simulink model "test_link_mux_demux"  (Simulink 7.3)
settings: Solver=ode45  StartTime=0.0  StopTime=100  RelTol=1e-3
undefined symbols (not defined in the file): ROACH
libraries: xbsIndex_r4 x46, xps_library x9, isi_correlator_lib x6, casper_library x1
settings Model: Creator=wjm  LastModifiedBy=wjm
settings OptimizationCC: InitFltsAndDblsToZero=on

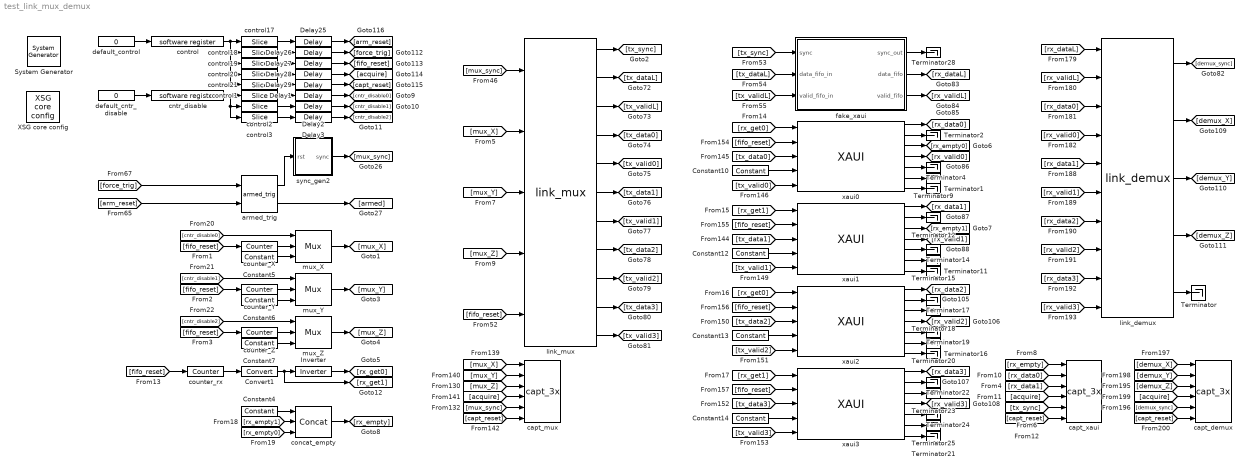
== system test_link_mux_demux ==
  " System Generator" : xbsIndex_r4/ System Generator  Tag=genX  SystemSampleTime=-1  xilinxfamily=virtex5  part=xc5vsx95t  speed=-1  package=ff1136  synthesis_tool=XST  clock_wrapper=Clock Enables  directory=./test_link_mux_demux/sysgen  testbench=off  simulink_period=1  sysclk_period=5  dcm_input_clock_period=100  incr_netlist=off  trim_vbits=Everywhere in SubSystem  dbl_ovrd=According to Block Masks  core_generation=According to Block Masks  run_coregen=off  deprecated_control=off  eval_field=0  block_type=sysgen
      settings: block_version=10.1.1
  Constant{10,12..14} (4 alike) : xbsIndex_r4/Constant  arith_type=Unsigned  const=0  n_bits=8  bin_pt=0  explicit_period=on  period=1  equ=P=C  opselect=C  inp2=PCIN>>17  opr=+  inp1=P  carry=CIN  dbl_ovrd=off  block_type=constant
      settings: block_version=10.1.1
  Constant{4..7} (4 alike) : xbsIndex_r4/Constant  arith_type=Unsigned  const=0  n_bits=30  bin_pt=0  explicit_period=on  period=1  equ=P=C  opselect=C  inp2=PCIN>>17  opr=+  inp1=P  carry=CIN  dbl_ovrd=off  block_type=constant
      settings: block_version=10.1.1
  Convert1 : xbsIndex_r4/Convert  arith_type=Boolean  n_bits=1  bin_pt=0  quantization=Truncate  overflow=Wrap  latency=3  dbl_ovrd=off  pipeline=on  block_type=convert
      settings: block_version=10.1.3
  Delay{1..3,25..29} (8 alike) : xbsIndex_r4/Delay  en=off  latency=3  dbl_ovrd=off  reg_retiming=off  block_type=delay
  Inverter : xbsIndex_r4/Inverter  en=off  latency=0  dbl_ovrd=off  block_type=inv
      settings: block_version=11.3
  Terminator{,1..2,4,9,11..12,14..25,28} (20 alike) : Terminator
  XSG core config : xps_library/XSG core config  Tag=xps:xsg  SystemSampleTime=-1  hw_sys=ROACH:sx95t  ibob_linux=off  clk_src=sys_clk2x  iBOB_clk_src=sys_clk  BEE2_ctrl_clk_src=sys_clk  BEE2_usr_clk_src=sys_clk  ROACH_clk_src=sys_clk2x  CORR_clk_src=sys_clk  gpio_clk_io_group=iBOB:sma  gpio_clk_bit_index=0  clk_rate=200  sample_period=1  synthesis_tool=XST  mpc_type=powerpc440_ext
  armed_trig : isi_correlator_lib/armed_trig  SystemSampleTime=-1
  capt_demux : isi_correlator_lib/capt_3x  SystemSampleTime=-1
      link override bram0/convert_din: arith_type=Unsigned
      link override bram0/mem/sim_data_in: arith_type=Unsigned
      link override bram0/test_link_mux_demux_capt_demux_bram0_data_out: arith_type=Unsigned
      link override bram1/convert_din: arith_type=Unsigned
      link override bram1/mem/sim_data_in: arith_type=Unsigned
      link override bram1/test_link_mux_demux_capt_demux_bram1_data_out: arith_type=Unsigned
      link override bram2/convert_din: arith_type=Unsigned
      link override bram2/mem/sim_data_in: arith_type=Unsigned
      link override bram2/test_link_mux_demux_capt_demux_bram2_data_out: arith_type=Unsigned
  capt_mux : isi_correlator_lib/capt_3x  SystemSampleTime=-1
      link override bram0/convert_din: arith_type=Unsigned
      link override bram0/mem/sim_data_in: arith_type=Unsigned
      link override bram0/test_link_mux_demux_capt_mux_bram0_data_out: arith_type=Unsigned
      link override bram1/convert_din: arith_type=Unsigned
      link override bram1/mem/sim_data_in: arith_type=Unsigned
      link override bram1/test_link_mux_demux_capt_mux_bram1_data_out: arith_type=Unsigned
      link override bram2/convert_din: arith_type=Unsigned
      link override bram2/mem/sim_data_in: arith_type=Unsigned
      link override bram2/test_link_mux_demux_capt_mux_bram2_data_out: arith_type=Unsigned
  capt_xaui : isi_correlator_lib/capt_3x  SystemSampleTime=-1
      link override bram0/convert_din: arith_type=Unsigned
      link override bram0/mem/sim_data_in: arith_type=Unsigned
      link override bram0/test_link_mux_demux_capt_demux_bram0_data_out: arith_type=Unsigned
      link override bram1/convert_din: arith_type=Unsigned
      link override bram1/mem/sim_data_in: arith_type=Unsigned
      link override bram1/test_link_mux_demux_capt_demux_bram1_data_out: arith_type=Unsigned
      link override bram2/convert_din: arith_type=Unsigned
      link override bram2/mem/sim_data_in: arith_type=Unsigned
      link override bram2/test_link_mux_demux_capt_demux_bram2_data_out: arith_type=Unsigned
  cntr_disable : xps_library/software register  Tag=xps:sw_reg  SystemSampleTime=-1  io_dir=From Processor  arith_type=Unsigned  bitwidth=32  bin_pt=0  sample_period=1  gw_name=test_link_mux_demux_cntr_disable_user_data_out
      link override corr_3ghz_10_1_corr_id_user_data_out: arith_type=Unsigned  n_bits=32  bin_pt=0  period=1
      link override corr_3ghz_10_1_exp_corr_id_user_data_out: arith_type=Unsigned  n_bits=32  bin_pt=0  period=1
      link override isi_corr_eq_coeff_user_data_out: arith_type=Unsigned  n_bits=32  bin_pt=0  period=1
      link override isi_correlator_control_user_data_out: arith_type=Unsigned  n_bits=32  bin_pt=0  period=1
      link override isi_correlator_cropped_control_user_data_out: arith_type=Unsigned  n_bits=32  bin_pt=0  period=1
      link override isi_correlator_eq_coeff_user_data_out: arith_type=Unsigned  n_bits=32  bin_pt=0  period=1
      link override isi_spectrometer_control_user_data_out: arith_type=Unsigned  n_bits=32  bin_pt=0  period=1
      link override isi_spectrometer_cropped_control_user_data_out: arith_type=Unsigned  n_bits=32  bin_pt=0  period=1
      link override isi_spectrometer_with_pfb_control_user_data_out: arith_type=Unsigned  n_bits=32  bin_pt=0  period=1
      link override roach_spectrometer_control_user_data_out: arith_type=Unsigned  n_bits=32  bin_pt=0  period=1
      link override test_link_mux_demux_control_user_data_out: arith_type=Unsigned  n_bits=32  bin_pt=0  period=1
  concat_empty : xbsIndex_r4/Concat  num_inputs=3  dbl_ovrd=off  block_type=concat
      settings: block_version=10.1.1
  control : xps_library/software register  Tag=xps:sw_reg  SystemSampleTime=-1  io_dir=From Processor  arith_type=Unsigned  bitwidth=32  bin_pt=0  sample_period=1  gw_name=test_link_mux_demux_control_user_data_out
      link override corr_3ghz_10_1_corr_id_user_data_out: arith_type=Unsigned  n_bits=32  bin_pt=0  period=1
      link override corr_3ghz_10_1_exp_corr_id_user_data_out: arith_type=Unsigned  n_bits=32  bin_pt=0  period=1
      link override isi_corr_eq_coeff_user_data_out: arith_type=Unsigned  n_bits=32  bin_pt=0  period=1
      link override isi_correlator_control_user_data_out: arith_type=Unsigned  n_bits=32  bin_pt=0  period=1
      link override isi_correlator_cropped_control_user_data_out: arith_type=Unsigned  n_bits=32  bin_pt=0  period=1
      link override isi_correlator_eq_coeff_user_data_out: arith_type=Unsigned  n_bits=32  bin_pt=0  period=1
      link override isi_spectrometer_control_user_data_out: arith_type=Unsigned  n_bits=32  bin_pt=0  period=1
      link override isi_spectrometer_cropped_control_user_data_out: arith_type=Unsigned  n_bits=32  bin_pt=0  period=1
      link override isi_spectrometer_with_pfb_control_user_data_out: arith_type=Unsigned  n_bits=32  bin_pt=0  period=1
      link override roach_spectrometer_control_user_data_out: arith_type=Unsigned  n_bits=32  bin_pt=0  period=1
      link override test_link_mux_demux_control_user_data_out: arith_type=Unsigned  n_bits=32  bin_pt=0  period=1
  control1 : xbsIndex_r4/Slice  nbits=1  boolean_output=off  mode=Lower Bit Location + Width  bit1=0  base1=MSB of Input  bit0=0  base0=LSB of Input  dbl_ovrd=off  block_type=slice
      settings: block_version=10.1.3
  control17 : xbsIndex_r4/Slice  nbits=1  boolean_output=on  mode=Lower Bit Location + Width  bit1=0  base1=MSB of Input  bit0=0  base0=LSB of Input  dbl_ovrd=off  block_type=slice
      settings: infoedit="Extracts a given range of bits from each input sample and presents it at the output.  The output type is ordinarily unsigned with binary point at zero, but can be Boolean when the slice is one bit wide.<P><P>Hardware notes: In hardware this block costs nothing."  block_version=10.1.3
  control18 : xbsIndex_r4/Slice  nbits=1  boolean_output=on  mode=Lower Bit Location + Width  bit1=0  base1=MSB of Input  bit0=1  base0=LSB of Input  dbl_ovrd=off  block_type=slice
      settings: infoedit="Extracts a given range of bits from each input sample and presents it at the output.  The output type is ordinarily unsigned with binary point at zero, but can be Boolean when the slice is one bit wide.<P><P>Hardware notes: In hardware this block costs nothing."  block_version=10.1.3
  control19 : xbsIndex_r4/Slice  nbits=1  boolean_output=on  mode=Lower Bit Location + Width  bit1=0  base1=MSB of Input  bit0=2  base0=LSB of Input  dbl_ovrd=off  block_type=slice
      settings: infoedit="Extracts a given range of bits from each input sample and presents it at the output.  The output type is ordinarily unsigned with binary point at zero, but can be Boolean when the slice is one bit wide.<P><P>Hardware notes: In hardware this block costs nothing."  block_version=10.1.3
  control2 : xbsIndex_r4/Slice  nbits=1  boolean_output=off  mode=Lower Bit Location + Width  bit1=0  base1=MSB of Input  bit0=1  base0=LSB of Input  dbl_ovrd=off  block_type=slice
      settings: block_version=10.1.3
  control20 : xbsIndex_r4/Slice  nbits=1  boolean_output=on  mode=Lower Bit Location + Width  bit1=0  base1=MSB of Input  bit0=3  base0=LSB of Input  dbl_ovrd=off  block_type=slice
      settings: infoedit="Extracts a given range of bits from each input sample and presents it at the output.  The output type is ordinarily unsigned with binary point at zero, but can be Boolean when the slice is one bit wide.<P><P>Hardware notes: In hardware this block costs nothing."  block_version=10.1.3
  control21 : xbsIndex_r4/Slice  nbits=1  boolean_output=on  mode=Lower Bit Location + Width  bit1=0  base1=MSB of Input  bit0=4  base0=LSB of Input  dbl_ovrd=off  block_type=slice
      settings: infoedit="Extracts a given range of bits from each input sample and presents it at the output.  The output type is ordinarily unsigned with binary point at zero, but can be Boolean when the slice is one bit wide.<P><P>Hardware notes: In hardware this block costs nothing."  block_version=10.1.3
  control3 : xbsIndex_r4/Slice  nbits=1  boolean_output=off  mode=Lower Bit Location + Width  bit1=0  base1=MSB of Input  bit0=2  base0=LSB of Input  dbl_ovrd=off  block_type=slice
      settings: block_version=10.1.3
  counter_X : xbsIndex_r4/Counter  cnt_type=Free Running  cnt_to=Inf  operation=Up  start_count=0  cnt_by_val=1  arith_type=Unsigned  n_bits=30  bin_pt=0  load_pin=off  rst=on  en=off  explicit_period=on  period=1  dbl_ovrd=off  use_behavioral_HDL=off  implementation=Fabric  use_rpm=off  block_type=counter
  counter_Y : xbsIndex_r4/Counter  cnt_type=Free Running  cnt_to=Inf  operation=Up  start_count=0  cnt_by_val=1  arith_type=Unsigned  n_bits=30  bin_pt=0  load_pin=off  rst=on  en=off  explicit_period=on  period=1  dbl_ovrd=off  use_behavioral_HDL=off  implementation=Fabric  use_rpm=off  block_type=counter
  counter_Z : xbsIndex_r4/Counter  cnt_type=Free Running  cnt_to=Inf  operation=Up  start_count=0  cnt_by_val=1  arith_type=Unsigned  n_bits=30  bin_pt=0  load_pin=off  rst=on  en=off  explicit_period=on  period=1  dbl_ovrd=off  use_behavioral_HDL=off  implementation=Fabric  use_rpm=off  block_type=counter
  counter_rx : xbsIndex_r4/Counter  cnt_type=Free Running  cnt_to=Inf  operation=Up  start_count=0  cnt_by_val=1  arith_type=Unsigned  n_bits=1  bin_pt=0  load_pin=off  rst=on  en=off  explicit_period=on  period=1  dbl_ovrd=off  use_behavioral_HDL=off  implementation=Fabric  use_rpm=off  block_type=counter
  default_cntr_disable : Constant  Value=0  OutDataType=sfix(16)  OutScaling=2^0  SampleTime=1
  default_control : Constant  Value=0  OutDataType=sfix(16)  OutScaling=2^0  SampleTime=1
  fake_xaui : Subsystem  AncestorBlock=isi_correlator_lib/fake_xaui  mask{latency=64}
  link_demux : isi_correlator_lib/link_demux  SystemSampleTime=-1  buffer_depth=8  logic_latency=1  mux_latency=1
  link_mux : isi_correlator_lib/link_mux  SystemSampleTime=-1
  mux_X : xbsIndex_r4/Mux  inputs=2  en=off  latency=0  precision=Full  arith_type=Unsigned  n_bits=16  bin_pt=14  quantization=Truncate  overflow=Wrap  dbl_ovrd=off  block_type=mux
      settings: block_version=11.3
  mux_Y : xbsIndex_r4/Mux  inputs=2  en=off  latency=0  precision=Full  arith_type=Unsigned  n_bits=16  bin_pt=14  quantization=Truncate  overflow=Wrap  dbl_ovrd=off  block_type=mux
      settings: block_version=11.3
  mux_Z : xbsIndex_r4/Mux  inputs=2  en=off  latency=0  precision=Full  arith_type=Unsigned  n_bits=16  bin_pt=14  quantization=Truncate  overflow=Wrap  dbl_ovrd=off  block_type=mux
      settings: block_version=11.3
  sync_gen2 : Subsystem  AncestorBlock=isi_correlator_lib/sync_gen2  mask(sync_gen2){using_pfb_fir=off, pfb_fir_taps=4, using_fft=off, fft_size=7, fft_inputs=4, fft_orders=[2 2 2 1], using_ct=off, ct_type=Double-buffered, using_vacc=off, vacc_length=0, using_scale_factor=on, scale_factor=2^20}
      mask prompts: using_pfb_fir "This design uses a PFB FIR."; pfb_fir_taps "Number of taps in PFB FIR:"; using_fft "This design uses an FFT."; fft_size "Size of FFT: (2^?)"; fft_inputs "Number of FFT inputs: (2^?)"; fft_orders "Order of FFT reorders: (vector)"; using_ct "This design uses a corner turner."; ct_type "Type of reorder operation:"; using_vacc "This design uses a vector accumulator."; vacc_length "Length of accumulations: (2^?)"; using_scale_factor "Scale the minimum period by an arbitrary amount."; scale_factor "Scale factor:"
      mask help: This block generates a sync pulse of an appropriate period based on the specified mask parameters.
      mask init:
      | sync_gen2_init(gcb, ...
      |     'using_pfb_fir', using_pfb_fir, ...
      |     'pfb_fir_taps', pfb_fir_taps, ...
      |     'using_fft', using_fft, ...
      |     'fft_size', fft_size, ...
      |     'fft_inputs', fft_inputs, ...
      |     'fft_orders', fft_orders, ...
      |     'using_ct', using_ct, ...
      |     'ct_type', ct_type, ...
      |     'using_vacc', using_vacc, ...
      |     'vacc_length', vacc_length, ...
      |     'using_scale_factor', using_scale_factor, ...
      |     'scale_factor', scale_factor);
      settings: AttributesFormatString=sync_period=1048576
      mask StyleString: checkbox,edit,checkbox,edit,edit,edit,checkbox,popup(Double-buffered|In-place),checkbox,edit,checkbox,edit
      mask CallbackString:
      | thisVariable = 'using_pfb_fir';
      | affectedVars = {'pfb_fir_taps'};
      | 
      | thisBlock = gcb();
      | thisVarState = get_param(thisBlock, thisVariable);
      | maskNames = get_param(thisBlock, 'MaskNames');
      | maskEnables = get_param(thisBlock, 'MaskEnables');
      | 
      | for varName = affectedVars
      |     varIndex = find(ismember(maskNames, varName));
      |     maskEnables{varIndex} = thisVarState;
      | end
      | 
      | set_param(thisBlock, 'MaskEnables', maskEnables);||thisVariable = 'using_fft';
      | affectedVars = {'fft_size', 'fft_inputs', 'fft_orders'};
      | 
      | thisBlock = gcb();
      | thisVarState = get_param(thisBlock, thisVariable);
      | maskNames = get_param(thisBlock, 'MaskNames');
      | maskEnables = get_param(thisBlock, 'MaskEnables');
      | 
      | for varName = affectedVars
      |     varIndex = find(ismember(maskNames, varName));
      |     maskEnables{varIndex} = thisVarState;
      | end
      | 
      | set_param(thisBlock, 'MaskEnables', maskEnables);||||thisVariable = 'using_ct';
      | affectedVars = {'ct_type'};
      | 
      | thisBlock = gcb();
      | thisVarState = get_param(thisBlock, thisVariable);
      | maskNames = get_param(thisBlock, 'MaskNames');
      | maskEnables = get_param(thisBlock, 'MaskEnables');
      | 
      | for varName = affectedVars
      |     varIndex = find(ismember(maskNames, varName));
      |     maskEnables{varIndex} = thisVarState;
      | end
      | 
      | set_param(thisBlock, 'MaskEnables', maskEnables);||thisVariable = 'using_vacc';
      | affectedVars = {'vacc_length'};
      | 
      | thisBlock = gcb();
      | thisVarState = get_param(thisBlock, thisVariable);
      | maskNames = get_param(thisBlock, 'MaskNames');
      | maskEnables = get_param(thisBlock, 'MaskEnables');
      | 
      | for varName = affectedVars
      |     varIndex = find(ismember(maskNames, varName));
      |     maskEnables{varIndex} = thisVarState;
      | end
      | 
      | set_param(thisBlock, 'MaskEnables', maskEnables);||thisVariable = 'using_scale_factor';
      | affectedVars = {'scale_factor'};
      | 
      | thisBlock = gcb();
      | thisVarState = get_param(thisBlock, thisVariable);
      | maskNames = get_param(thisBlock, 'MaskNames');
      | maskEnables = get_param(thisBlock, 'MaskEnables');
      | 
      | for varName = affectedVars
      |     varIndex = find(ismember(maskNames, varName));
      |     maskEnables{varIndex} = thisVarState;
      | end
      | 
      | set_param(thisBlock, 'MaskEnables', maskEnables);|
  xaui0 : xps_library/XAUI  Tag=xps:xaui  SystemSampleTime=-1  demux=2  port=ROACH:0  open_phy=on  show_param=off  pre_emph=3  swing=800
      link override convert_tx_data: n_bits=32
      link override convert_tx_outofband: n_bits=4
      link override test_link_mux_demux_xaui0_rx_data: n_bits=32
      link override test_link_mux_demux_xaui0_rx_outofband: n_bits=4
  xaui1 : xps_library/XAUI  Tag=xps:xaui  SystemSampleTime=-1  demux=2  port=ROACH:1  open_phy=on  show_param=off  pre_emph=3  swing=800
      link override convert_tx_data: n_bits=32
      link override convert_tx_outofband: n_bits=4
      link override test_link_mux_demux_xaui1_rx_data: n_bits=32
      link override test_link_mux_demux_xaui1_rx_outofband: n_bits=4
  xaui2 : xps_library/XAUI  Tag=xps:xaui  SystemSampleTime=-1  demux=2  port=ROACH:2  open_phy=on  show_param=off  pre_emph=3  swing=800
      link override convert_tx_data: n_bits=32
      link override convert_tx_outofband: n_bits=4
      link override test_link_mux_demux_xaui2_rx_data: n_bits=32
      link override test_link_mux_demux_xaui2_rx_outofband: n_bits=4
  xaui3 : xps_library/XAUI  Tag=xps:xaui  SystemSampleTime=-1  demux=2  port=ROACH:3  open_phy=on  show_param=off  pre_emph=3  swing=800
      link override convert_tx_data: n_bits=32
      link override convert_tx_outofband: n_bits=4
      link override test_link_mux_demux_xaui3_rx_data: n_bits=32
      link override test_link_mux_demux_xaui3_rx_outofband: n_bits=4
  wires:
  [mux_X] -> capt_mux/1
  [mux_Y] -> capt_mux/2
  [mux_Z] -> capt_mux/3
  [capt_reset] -> capt_mux/6
  [fifo_reset] -> link_mux/5
  link_mux/1 -> [tx_sync]
  link_mux/2 -> [tx_dataL]
  link_mux/3 -> [tx_validL]
  link_mux/4 -> [tx_data0]
  link_mux/5 -> [tx_valid0]
  link_mux/6 -> [tx_data1]
  link_mux/7 -> [tx_valid1]
  link_mux/8 -> [tx_data2]
  link_mux/9 -> [tx_valid2]
  link_mux/10 -> [tx_data3]
  link_mux/11 -> [tx_valid3]
  [tx_sync] -> fake_xaui/1(sync)
  [tx_dataL] -> fake_xaui/2(data_fifo_in)
  [tx_validL] -> fake_xaui/3(valid_fifo_in)
  [fifo_reset] -> xaui0/2
  [tx_data0] -> xaui0/3
  Constant10/1 -> xaui0/4
  [tx_valid0] -> xaui0/5
  [fifo_reset] -> xaui1/2
  [tx_data1] -> xaui1/3
  Constant12/1 -> xaui1/4
  [tx_valid1] -> xaui1/5
  [fifo_reset] -> xaui2/2
  [tx_data2] -> xaui2/3
  Constant13/1 -> xaui2/4
  [tx_valid2] -> xaui2/5
  [fifo_reset] -> xaui3/2
  [tx_data3] -> xaui3/3
  Constant14/1 -> xaui3/4
  [tx_valid3] -> xaui3/5
  xaui0/1 -> [rx_data0]
  xaui0/2 -> Terminator2/1
  xaui0/3 -> [rx_empty0]
  xaui0/4 -> [rx_valid0]
  xaui0/5 -> Terminator4/1
  xaui0/6 -> Terminator9/1
  xaui0/7 -> Terminator1/1
  xaui1/1 -> [rx_data1]
  xaui1/2 -> Terminator12/1
  xaui1/3 -> [rx_empty1]
  xaui1/4 -> [rx_valid1]
  xaui1/5 -> Terminator14/1
  xaui1/6 -> Terminator15/1
  xaui1/7 -> Terminator11/1
  xaui2/1 -> [rx_data2]
  xaui2/2 -> Terminator17/1
  xaui2/3 -> Terminator18/1
  xaui2/4 -> [rx_valid2]
  xaui2/5 -> Terminator19/1
  xaui2/6 -> Terminator20/1
  xaui2/7 -> Terminator16/1
  xaui3/1 -> [rx_data3]
  xaui3/2 -> Terminator22/1
  xaui3/3 -> Terminator23/1
  xaui3/4 -> [rx_valid3]
  xaui3/5 -> Terminator24/1
  xaui3/6 -> Terminator25/1
  xaui3/7 -> Terminator21/1
  fake_xaui/2(data_fifo) -> [rx_dataL]
  fake_xaui/3(valid_fifo) -> [rx_validL]
  [acquire] -> capt_mux/4
  [mux_sync] -> capt_mux/5
  fake_xaui/1(sync_out) -> Terminator28/1
  [demux_Y] -> capt_demux/2
  [demux_Z] -> capt_demux/3
  [capt_reset] -> capt_demux/6
  [acquire] -> capt_demux/4
  [demux_sync] -> capt_demux/5
  [arm_reset] -> armed_trig/2
  [force_trig] -> armed_trig/1
  armed_trig/1 -> sync_gen2/1(rst)
  armed_trig/2 -> [armed]
  sync_gen2/1(sync) -> [mux_sync]
  control21/1 -> Delay29/1
  control20/1 -> Delay28/1
  control19/1 -> Delay27/1
  control18/1 -> Delay26/1
  control17/1 -> Delay25/1
  control/1 -> control17/1, control18/1, control19/1, control21/1, control20/1
  Delay26/1 -> [force_trig]
  Delay27/1 -> [fifo_reset]
  Delay28/1 -> [acquire]
  Delay29/1 -> [capt_reset]
  default_control/1 -> control/1
  Delay25/1 -> [arm_reset]
  [mux_sync] -> link_mux/1
  [rx_dataL] -> link_demux/1
  [rx_validL] -> link_demux/2
  [rx_data0] -> link_demux/3
  [rx_valid0] -> link_demux/4
  [rx_data1] -> link_demux/5
  [rx_valid1] -> link_demux/6
  [rx_data2] -> link_demux/7
  [rx_valid2] -> link_demux/8
  [rx_data3] -> link_demux/9
  [rx_valid3] -> link_demux/10
  link_demux/5 -> Terminator/1
  link_demux/4 -> [demux_Z]
  link_demux/3 -> [demux_Y]
  link_demux/2 -> [demux_X]
  link_demux/1 -> [demux_sync]
  [demux_X] -> capt_demux/1
  [fifo_reset] -> counter_X/1
  [fifo_reset] -> counter_Y/1
  [fifo_reset] -> counter_Z/1
  [rx_data0] -> capt_xaui/2
  [rx_data1] -> capt_xaui/3
  [capt_reset] -> capt_xaui/6
  [acquire] -> capt_xaui/4
  [tx_sync] -> capt_xaui/5
  [rx_empty] -> capt_xaui/1
  [fifo_reset] -> counter_rx/1
  counter_rx/1 -> Convert1/1
  [rx_get0] -> xaui0/1
  [rx_get1] -> xaui1/1
  [rx_get0] -> xaui2/1
  [rx_get1] -> xaui3/1
  Constant4/1 -> concat_empty/1
  [rx_empty1] -> concat_empty/2
  [rx_empty0] -> concat_empty/3
  concat_empty/1 -> [rx_empty]
  default_cntr_disable/1 -> cntr_disable/1
  mux_X/1 -> [mux_X]
  mux_Y/1 -> [mux_Y]
  mux_Z/1 -> [mux_Z]
  counter_Z/1 -> mux_Z/2
  Constant7/1 -> mux_Z/3
  Constant6/1 -> mux_Y/3
  counter_Y/1 -> mux_Y/2
  Constant5/1 -> mux_X/3
  counter_X/1 -> mux_X/2
  cntr_disable/1 -> control1/1, control3/1, control2/1
  control1/1 -> Delay1/1
  Delay1/1 -> [cntr_disable0]
  [cntr_disable0] -> mux_X/1
  [cntr_disable1] -> mux_Y/1
  [cntr_disable2] -> mux_Z/1
  Convert1/1 -> Inverter/1, [rx_get1]
  control2/1 -> Delay2/1
  Delay2/1 -> [cntr_disable1]
  control3/1 -> Delay3/1
  Delay3/1 -> [cntr_disable2]
  [mux_Y] -> link_mux/3
  [mux_Z] -> link_mux/4
  [mux_X] -> link_mux/2
  Inverter/1 -> [rx_get0]

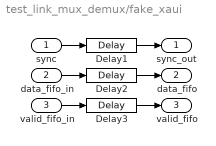
== system test_link_mux_demux/fake_xaui ==
  sync : Inport  OutDataType=sfix(16)  OutScaling=2^0
  data_fifo_in : Inport  Port=2  OutDataType=sfix(16)  OutScaling=2^0
  valid_fifo_in : Inport  Port=3  OutDataType=sfix(16)  OutScaling=2^0
  Delay1 : xbsIndex_r4/Delay  en=off  latency=latency  dbl_ovrd=off  reg_retiming=off  block_type=delay
  Delay2 : xbsIndex_r4/Delay  en=off  latency=latency  dbl_ovrd=off  reg_retiming=off  block_type=delay
  Delay3 : xbsIndex_r4/Delay  en=off  latency=latency  dbl_ovrd=off  reg_retiming=off  block_type=delay
  sync_out : Outport  OutDataType=sfix(16)  OutScaling=2^0
  data_fifo : Outport  Port=2  OutDataType=sfix(16)  OutScaling=2^0
  valid_fifo : Outport  Port=3  OutDataType=sfix(16)  OutScaling=2^0
  wires:
  valid_fifo_in/1 -> Delay3/1
  data_fifo_in/1 -> Delay2/1
  sync/1 -> Delay1/1
  Delay1/1 -> sync_out/1
  Delay2/1 -> data_fifo/1
  Delay3/1 -> valid_fifo/1

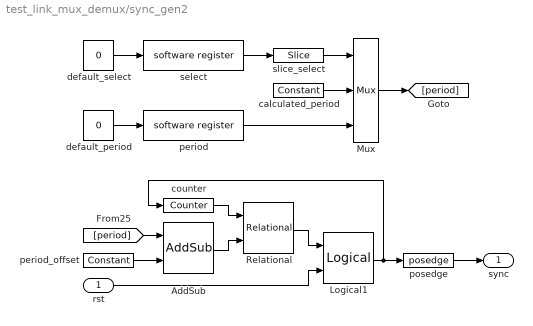
== system test_link_mux_demux/sync_gen2 ==
  rst : Inport  OutDataType=sfix(16)  OutScaling=2^0
  AddSub : xbsIndex_r4/AddSub  mode=Subtraction  use_carryin=off  use_carryout=off  en=off  latency=2  precision=Full  arith_type=Unsigned  n_bits=16  bin_pt=14  quantization=Truncate  overflow=Wrap  dbl_ovrd=off  use_behavioral_HDL=off  hw_selection=Fabric  pipelined=off  use_rpm=on  block_type=addsub
      settings: block_version=10.1.3
  Logical1 : xbsIndex_r4/Logical  logical_function=OR  inputs=2  en=off  latency=0  precision=Full  arith_type=Unsigned  n_bits=16  bin_pt=0  align_bp=on  dbl_ovrd=off  block_type=logical
  Mux : xbsIndex_r4/Mux  inputs=2  en=off  latency=0  precision=Full  arith_type=Unsigned  n_bits=16  bin_pt=14  quantization=Truncate  overflow=Wrap  dbl_ovrd=off  block_type=mux
  Relational : xbsIndex_r4/Relational  mode=a>=b  en=off  latency=1  dbl_ovrd=off  block_type=relational
      settings: block_version=10.1.3
  calculated_period : xbsIndex_r4/Constant  arith_type=Unsigned  const=1048576  n_bits=32  bin_pt=0  explicit_period=on  period=1  equ=P=C  opselect=C  inp2=PCIN>>17  opr=+  inp1=P  carry=CIN  dbl_ovrd=off  block_type=constant
      settings: block_version=10.1.1
  counter : xbsIndex_r4/Counter  cnt_type=Free Running  cnt_to=Inf  operation=Up  start_count=0  cnt_by_val=1  arith_type=Unsigned  n_bits=32  bin_pt=0  load_pin=off  rst=on  en=off  explicit_period=on  period=1  dbl_ovrd=off  use_behavioral_HDL=off  implementation=Fabric  use_rpm=off  block_type=counter
  default_period : Constant  Value=0  OutDataType=sfix(16)  OutScaling=2^0  SampleTime=1
  default_select : Constant  Value=0  OutDataType=sfix(16)  OutScaling=2^0  SampleTime=1
  period : xps_library/software register  Tag=xps:sw_reg  SystemSampleTime=-1  io_dir=From Processor  arith_type=Unsigned  bitwidth=32  bin_pt=0  sample_period=1  gw_name=test_link_mux_demux_sync_gen2_period_user_data_out
      link override test_link_mux_demux_sync_gen2_period_user_data_out: arith_type=Unsigned  n_bits=32  bin_pt=0  period=1
  period_offset : xbsIndex_r4/Constant  arith_type=Unsigned  const=3  n_bits=32  bin_pt=0  explicit_period=on  period=1  equ=P=C  opselect=C  inp2=PCIN>>17  opr=+  inp1=P  carry=CIN  dbl_ovrd=off  block_type=constant
      settings: block_version=10.1.1
  posedge : casper_library/Misc/posedge  Tag=Rising Edge Detector  SystemSampleTime=-1
  select : xps_library/software register  Tag=xps:sw_reg  SystemSampleTime=-1  io_dir=From Processor  arith_type=Unsigned  bitwidth=32  bin_pt=0  sample_period=1  gw_name=test_link_mux_demux_sync_gen2_select_user_data_out
      link override test_link_mux_demux_sync_gen2_select_user_data_out: arith_type=Unsigned  n_bits=32  bin_pt=0  period=1
  slice_select : xbsIndex_r4/Slice  nbits=1  boolean_output=on  mode=Lower Bit Location + Width  bit1=0  base1=MSB of Input  bit0=0  base0=LSB of Input  dbl_ovrd=off  block_type=slice
      settings: infoedit="Extracts a given range of bits from each input sample and presents it at the output.  The output type is ordinarily unsigned with binary point at zero, but can be Boolean when the slice is one bit wide.<P><P>Hardware notes: In hardware this block costs nothing."  block_version=10.1.3
  sync : Outport  OutDataType=sfix(16)  OutScaling=2^0
  wires:
  Mux/1 -> [period]
  period/1 -> Mux/3
  calculated_period/1 -> Mux/2
  slice_select/1 -> Mux/1
  default_period/1 -> period/1
  select/1 -> slice_select/1
  default_select/1 -> select/1
  [period] -> AddSub/1
  period_offset/1 -> AddSub/2
  AddSub/1 -> Relational/2
  counter/1 -> Relational/1
  Logical1/1 -> posedge/1, counter/1
  posedge/1 -> sync/1
  Relational/1 -> Logical1/1
  rst/1 -> Logical1/2
